simulink model "dspmrf_wlp"  (Simulink 5.0)
settings: Solver=FixedStepDiscrete  SolverMode=SingleTasking  StartTime=0.0  StopTime=inf  RelTol=1e-3  AbsTol=1e-6
PreLoadFcn:
  | load dspmrf_coeffs
values from neighbouring files (symbols this model uses):
  mrf_firdn1 = [-6.50674965731e-05 -2.86394301669e-05 -3.28947367672e-05 -3.58831696283e-05 -3.71134312214e-05 -3.60823694959e-05 -3.23581725714e-05 -2.55641169189e-05 -1.5457983534e-05 -1.90570408935e-06 1.50461966328e-05 3.52080664946e-05 ... (685 elements, 1x685)]    [dspmrf_coeffs.mat]
  mrf_upfir1 = [-0.000780809958877 -0.000343673162003 -0.000394736841206 -0.000430598035539 -0.000445361174657 -0.000432988433951 -0.000388298070857 -0.000306769403027 -0.000185495802408 -2.28684490722e-05 0.000180554359593 0.000422496797935 ... (685 elements, 1x685)]    [dspmrf_coeffs.mat]
libraries: dspmlti3 x4, dspsigops x1, dspsrcs4 x1, dspmrf_lib x1
settings Model: Creator=don  LastModifiedBy=mkhan  ExtModeTrigMode=oneshot  ExtModeArmWhenConnect=off  SaveTime=off  SaveOutput=off  LimitDataPoints=off  IntegerOverflowMsg=none  BlockReductionOpt=off  BooleanDataType=off  ZeroCrossControl=UseLocalSettings  TargetHWChar=2  TargetHWWordLengths=8,16,32,32  RTWMathFcnLibMatFile=iso_c_tmw.mat  RTWOptions="-aEnforceIntegerDowncast=1 -aFoldNonRolledExpr=1 -aInlineInvariantSignals=1 -aInlineParameters=0 -aLocalBlockOutputs=1 -aRollThreshold=2 -aRTWVerbose=1 -aForceParamTrailComments=0 -aGenerateComments=1 -aIgnoreCustomStorageClasses=1 -aIncHierarchyInIds=0 -aMaxRTWIdLen=31 -aShowEliminatedStatements=0 -aReadOnly=0 -aTargetFcnLib=\"iso_c_tmw.mat\" -aIncDataTypeInIds=0 -aPrefixModelToSubsysFcnNames=1 -aInlinedPrmAccess=\"Literals\" -aGenerateFullHeader=1 -aIsPILTarget=0 -aGenerateReport=0 -aLogVarNameModifier=\"rt_\" -aExtMode=0 -aExtModeStaticAlloc=0 -aExtModeTesting=0 -aExtModeStaticAllocSize=1000000 -aExtModeTransport=0"

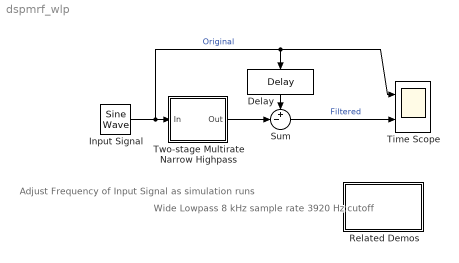
== system dspmrf_wlp ==
  note: Wide Lowpass
      | 8 kHz sample rate
      | 3920 Hz cutoff
  note: Adjust Frequency
      | of Input Signal
      | as simulation runs
  Delay : dspsigops/Delay  Orientation=down  dly_unit=Samples  delay=6096  ic_detail=on  dif_ic_for_ch=off  dif_ic_for_dly=off  ic=0  reset_popup=None
  Input Signal : dspsrcs4/Sine Wave  Amplitude=1  Frequency=4000-80  Phase=0  SampleMode=Discrete  OutComplex=Real  CompMethod=Trigonometric fcn  TableSize=Speed  SampleTime=1/8000  SamplesPerFrame=1  dataType=double  wordLen=16  udDataType=sfix(16)  fracBitsMode=Best precision  numFracBits=14  ResetState=Restart at time zero
  Related Demos : Subsystem
      settings: OpenFcn=dspmrf_menu
      mask Display: disp('Other\nMultirate Filter\nDemos')
  Sum : Sum  Inputs=+-|  SaturateOnIntegerOverflow=on  InputSameDT=on
  Time Scope : Scope  NumInputPorts=2
      settings: TimeRange=1.5  YMin=-2~-1.5  YMax=2~1.5  DataFormat=Structure
  Two-stage Multirate Narrow Highpass : Subsystem
  wires:
  Input Signal/1 -> Two-stage Multirate Narrow Highpass/1(In), Time Scope/1, Delay/1  "Original"
  Delay/1 -> Sum/1
  Two-stage Multirate Narrow Highpass/1(Out) -> Sum/2
  Sum/1 -> Time Scope/2  "Filtered"

== system dspmrf_wlp/Related Demos ==

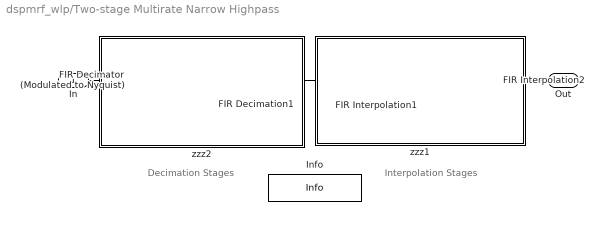
== system dspmrf_wlp/Two-stage Multirate Narrow Highpass ==
  note: Interpolation Stages
  note: Decimation Stages
  In : Inport
  FIR Decimation1 : dspmlti3/FIR Decimation  h=mrf_firdn2  D=4  framing=Maintain input frame size  outputBufInitCond=0
  FIR Interpolation1 : dspmlti3/FIR Interpolation  h=mrf_upfir2  L=4  framing=Maintain input frame size  outputBufInitCond=0
  FIR Interpolation2 : dspmlti3/FIR Interpolation  h=mrf_upfir1 .* ((-1).^(0:684))  L=12  framing=Maintain input frame size  outputBufInitCond=0
  FIR Decimator (Modulated to Nyquist) : dspmlti3/FIR Decimation  h=mrf_firdn1 .* ((-1).^(0:684))  D=12  framing=Maintain input frame size  outputBufInitCond=0
  Info : dspmrf_lib/Info
  zzz1 : Subsystem
      settings: OpenFcn=dspmsmrff;
      mask Display: disp('')
  zzz2 : Subsystem
      settings: OpenFcn=dspmsmrff;
      mask Display: disp('')
  Out : Outport
  wires:
  FIR Interpolation2/1 -> Out/1
  FIR Interpolation1/1 -> FIR Interpolation2/1
  FIR Decimation1/1 -> FIR Interpolation1/1
  FIR Decimator (Modulated to Nyquist)/1 -> FIR Decimation1/1
  In/1 -> FIR Decimator (Modulated to Nyquist)/1

== system dspmrf_wlp/Two-stage Multirate Narrow Highpass/zzz1 ==

== system dspmrf_wlp/Two-stage Multirate Narrow Highpass/zzz2 ==
